simulink model "aerosonde_controlled"  (Simulink 7.7)
settings: Solver=ode3  StartTime=0.0  StopTime=200  FixedStep=20e-3  RelTol=1e-6
values from neighbouring files (symbols this model uses):
  aerosonde = aerosonde_data    [aerosonde_initialize.m]    (also in aerosonde_trimlin.m)
  chi_trim = 0    [aerosonde_initialize.m]
  eta_trim = -0.1    [aerosonde_initialize.m]
  euler_0 = [theta_trim; 0; 0]    [aerosonde_initialize.m]    (also in aerosonde_trimlin.m = xtrim(11:13))
  flap = 0    [aerosonde_initialize.m]
  fuel_0 = 2    [aerosonde_initialize.m]    (also in aerosonde_trimlin.m = xtrim(10))
  h_trim = 500    [aerosonde_initialize.m]
  ignition = 1    [aerosonde_initialize.m]
  Kari = 0.5    [aerosonde_initialize.m]
  Kd_Ye = 0.6    [aerosonde_initialize.m]
  Kd_Ze = -0.05    [aerosonde_initialize.m]
  Ki_phi = -0.1    [aerosonde_initialize.m]
  Ki_psi = 0.001    [aerosonde_initialize.m]
  Ki_theta = -0.8    [aerosonde_initialize.m]
  Ki_u = 0.15    [aerosonde_initialize.m]
  Ki_Ye = 0.0025    [aerosonde_initialize.m]
  Ki_Ze = -0.0001    [aerosonde_initialize.m]
  Kp_phi = -0.2    [aerosonde_initialize.m]
  Kp_psi = 0.7    [aerosonde_initialize.m]
  Kp_theta = -0.8    [aerosonde_initialize.m]
  Kp_u = 0.5    [aerosonde_initialize.m]
  Kp_Xe = 0.125    [aerosonde_initialize.m]
  Kp_Ye = 0.18    [aerosonde_initialize.m]
  Kp_Ze = -0.03    [aerosonde_initialize.m]
  Kphi_xi = -0.2    [aerosonde_initialize.m]
  Kq_eta = -0.28    [aerosonde_initialize.m]
  Kr_zeta = -0.25    [aerosonde_initialize.m]
  Ktheta_eta = -1    [aerosonde_initialize.m]
  latitude = 52.073105    [aerosonde_initialize.m]
  longitude = -000.616697    (= -0.616697)    [aerosonde_initialize.m]
  mixture = 13    [aerosonde_initialize.m]
  Omega_0 = 5000*pi/30    (= 523.598775598)    [aerosonde_initialize.m]    (also in aerosonde_trimlin.m = xtrim(14))
  position_0 = [0; 0; -h_trim]    [aerosonde_initialize.m]
  q_trim = 0    [aerosonde_initialize.m]
  rates_0 = [0; q_trim ; 0]    [aerosonde_initialize.m]    (also in aerosonde_trimlin.m = xtrim(7:9))
  tau_trim = 0.4    [aerosonde_initialize.m]
  theta_trim = 0    [aerosonde_initialize.m]
  Tr = 0.75    [aerosonde_initialize.m]
  Ue_VL = 25    [aerosonde_initialize.m]
  Ve_VL = 0    [aerosonde_initialize.m]
  velocity_0 = [23; 0; 0]    [aerosonde_initialize.m]    (also in aerosonde_trimlin.m = xtrim(1:3))
  We_VL = 0    [aerosonde_initialize.m]
  Xe0_VL = position_0(1)    [aerosonde_initialize.m]
  xi_trim = 0    [aerosonde_initialize.m]
  Ye0_VL = position_0(2)    [aerosonde_initialize.m]
  Ze0_VL = position_0(3)    [aerosonde_initialize.m]
  zeta_trim = 0    [aerosonde_initialize.m]
undefined symbols (not defined in the file or in its folder): Earth, F, m, MIL, rad, s, WGS84
libraries: aerolibasang x4, aerolibbdyn x3, aerolibfltsims x3, simulink_extras x3, aerolibwind2 x3, aerolibtransform2 x2, aerolibatmos2 x2, aerolibconvert2 x2, simulink x2, aerolibadyn x1, aerolib6dof2 x1, aerolibutil x1
(part 1 of 2)
settings Model: Creator=eh3081  LastModifiedBy=eh3081
settings DataIOCC: LimitDataPoints=off  SaveOutput=off  SignalLogging=off  SaveTime=off
settings OptimizationCC: InitFltsAndDblsToZero=on
settings DebuggingCC: SaveWithParameterizedLinksMsg=none  MultiTaskDSMMsg=warning  MultiTaskCondExecSysMsg=none  StrictBusMsg=Warning
settings RTWCC: IncludeERTFirstTime=on
settings GRTTargetCC: TargetFcnLib=ansi_tfl_tmw.mat

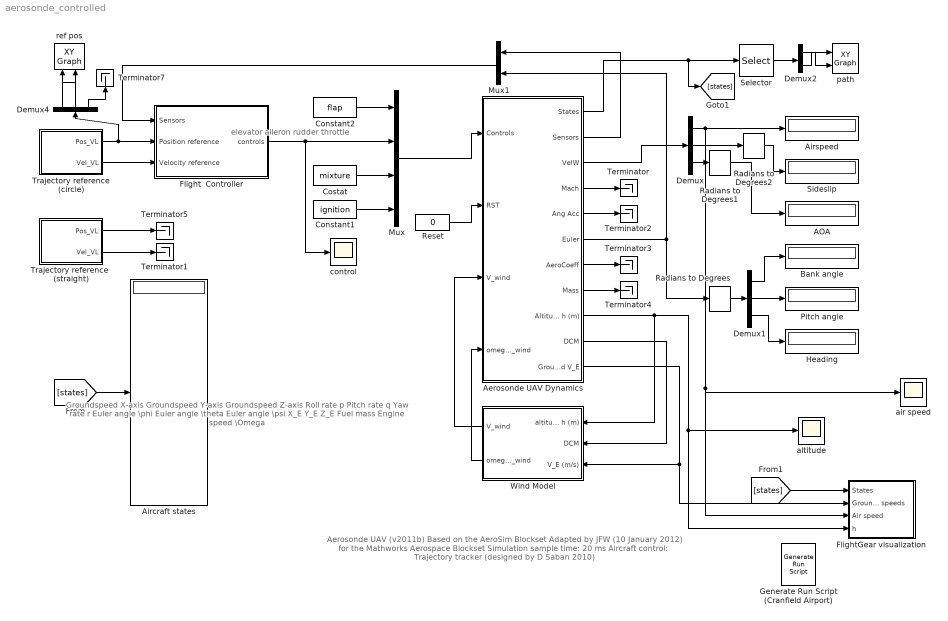
== system aerosonde_controlled ==
  note: Aerosonde UAV (v2011b)
      | Based on the AeroSim Blockset
      | Adapted by JFW (10 January 2012) for the Mathworks Aerospace Blockset
      | Simulation sample time: 20 ms
      | Aircraft control: Trajectory tracker (designed by D Saban 2010)
  note: Groundspeed X-axis
      | Groundspeed Y-axis
      | Groundspeed Z-axis
      | Roll rate p
      | Pitch rate q
      | Yaw rate r
      | Euler angle \phi
      | Euler angle \theta
      | Euler angle \psi
      | X_E
      | Y_E
      | Z_E
      | Fuel mass
      | Engine speed \Omega
  note: elevator
      | aileron
      | rudder
      | throttle
  AOA : Display
  Aerosonde UAV Dynamics : Subsystem  mask(6-DOF Aerosonde Model){as=aerosonde, Velocities0=velocity_0, Rates0=rates_0, Euler0=euler_0, Position0=position_0, Fuel0=fuel_0, Omega0=Omega_0, GndAlt=0}
      mask prompts: as "Aircraft configuration data:"; Velocities0 "Initial velocity in body axes [u,v,w]: (m/s)"; Rates0 "Initial body rotation rates [p,q,r]: (rad/s)"; Euler0 "Initial Euler orientation [roll, pitch, yaw]: (rad)"; Position0 "Initial position in inertial axes [Xe,Ye,Ze]: (m)"; Fuel0 "Initial fuel mass: (Kg)"; Omega0 "Initial engine speed: (rad/s)"; GndAlt "Ground altitude: (m)"
      mask help:
      | Nonlinear 6-DOF Aerosonde  model with equations of motion in
      | body frame.
      |
      | Version 2011a (18 February 2011)
      mask Help:
      | The block implements the 6-DOF nonlinear Aerosonde model. It is an adaptation of the model provided in the AeroSim blockset. Velocities are computed in body frame.
      | <P><B>Inputs:</B>
      | <LI>Controls = the 4x1 vector of aircraft controls [elevator aileron rudder throttle]. Aerodynamic controls are in radians, throttle is from 0 to 1.</LI>
      | <LI>RST = the integrator reset flag (0 or 1, all integrators on rising edge)
      | <LI>V_wind = the 3x1 vector of background wind speed components in navigation frame [North East Down]</LI>
      | <LI>omega_wind = the 3x1 vector of background wind angular rates in navigation frame [North East Down]</LI>
      | </P>
      | <P><B>Outputs:</B>
      | <LI>States = the 14x1 aircraft state vector [Velocities, Angular rates, Euler angles, Position, Fuel mass, Engine speed].</LI>
      | <LI>Sensors = the 15x1 vector of sensor outputs [GPS Position, GPS Groundspeed, Accelerometers, Gyros, Air data].</LI>
      | <LI>VelW = the 3x1 vector of aircraft velocity in wind axes [Airspeed, sideslip, angle of attack]</LI>
      | <LI>Mach = the Mach number</LI>
      | <LI>Ang Acc = the 3x1 vector of angular accelerations
      | <LI>Euler = the 3x1 vector of Euler angles (roll, pitch, yaw)</LI>
      | <LI>AeroCoeff = the 6x1 vector of aerodynamic coefficients [CD CY CL Cl Cm Cn]</LI>
      | <LI>Mass = the current aircraft mass</LI>
      | <LI>h = the aircraft altitude</LI>
      | </P>
      | <P><B>Parameters:</B>
      | <LI>Aircraft configuration data = structured varaible with aircraft data<BR>
      | obtain by  ``aerosonde=aerosonde_initialize'' for example</LI>
      | <LI>Initial velocities = the 3x1 vector of initial aircraft velocities in body axes [u v w]</LI>
      | <LI>Initial angular rates = the 3x1 vector of initial angular rates [p q r]</LI>
      | <LI>Initial attitude = the 3x1 vector of initial Euler angles [phi theta psi]</LI>
      | <LI>Initial position = the 3x1 vector of initial aircraft location [Lat Lon Alt]</LI>
      | <LI>Initial fuel mass = the initial quantity of fuel on-board the aircraft</LI>
      | <LI>Initial engine speed = the initial engine rotation speed</LI>
      | <LI>Ground altitude = the ground altitude at aircraft location</LI>
      | </P>
      | <P>
      | <I>Version 2010b (26 May 2010)</I>
      | </P>
  Aircraft states : Display
  Airspeed : Display
  Bank angle : Display
  Constant1 : Constant  Value=ignition
  Constant2 : Constant  Value=flap
  Costat : Constant  Value=mixture
  Demux : Demux  Outputs=3
  Demux1 : Demux  Outputs=3
  Demux2 : Demux  Outputs=2
  Demux4 : Demux  Outputs=3
  Flight  Controller : Subsystem
  FlightGear visualization : Subsystem  TreatAsAtomicUnit=on
  Generate Run Script (Cranfield Airport) : aerolibfltsims/Generate Run Script  SystemSampleTime=-1  OutputFileName=runfg.bat  FlightGearBaseDirectory=C:\Program Files\FlightGear 2.4.0  GeometryModelName=Aerosonde  DestinationPort=5502  AirportId=EGTC  RunwayId=3  InitialAltitude=h_trim*3.28083  InitialHeading=0  OffsetDistance=4.72  OffsetAzimuth=0  GenerateFile=off
  Heading : Display
  Mux : Mux  Inputs=[1 4 1 1]
  Mux1 : Mux  Inputs=[15 3]
  Pitch angle : Display
  Radians to Degrees : simulink_extras/Transformations/Radians to Degrees  SystemSampleTime=-1
  Radians to Degrees1 : simulink_extras/Transformations/Radians to Degrees  SystemSampleTime=-1
  Radians to Degrees2 : simulink_extras/Transformations/Radians to Degrees  SystemSampleTime=-1
  Reset : Constant  Value=0
  Selector : Selector  InputPortWidth=14  IndexOptions=Index vector (dialog)  Indices=[10 11]  OutputSizes=1
  Sideslip : Display
  Terminator{,1..5,7} (7 alike) : Terminator
  Trajectory reference (circle) : Subsystem
  Trajectory reference  (straight) : Subsystem
  Wind Model : Subsystem
  air speed : Scope
      settings: YMin=-2.5  YMax=25  SaveName=ScopeData2
  altitude : Scope
      settings: YMin=800  YMax=1025
  control : Scope
      settings: YMin=-0.1  YMax=1  SaveName=ScopeData5
  path : simulink/Sinks/XY Graph  SystemSampleTime=-1  xmin=-1000  xmax=1000  ymin=-1000  ymax=1000  st=-1
  ref pos : simulink/Sinks/XY Graph  SystemSampleTime=-1  xmin=-1000  xmax=1000  ymin=-1000  ymax=1000  st=-1
  wires:
  Reset/1 -> Aerosonde UAV Dynamics/2(RST)
  Aerosonde UAV Dynamics/1(States) -> Selector/1, [states]
  Aerosonde UAV Dynamics/6(Euler) -> Mux1/2, Radians to Degrees/1
  Demux/3 -> Radians to Degrees1/1
  Demux/2 -> Radians to Degrees2/1
  Demux/1 -> Airspeed/1, air speed/1, FlightGear visualization/3(Air speed)
  Radians to Degrees2/1 -> Sideslip/1
  Radians to Degrees1/1 -> AOA/1
  Radians to Degrees/1 -> Demux1/1
  Demux1/2 -> Pitch angle/1
  Demux1/3 -> Heading/1
  Demux1/1 -> Bank angle/1
  Aerosonde UAV Dynamics/3(VelW) -> Demux/1
  Wind Model/1(V_wind) -> Aerosonde UAV Dynamics/3(V_wind)
  Wind Model/2(omega_wind) -> Aerosonde UAV Dynamics/4(omega_wind)
  Aerosonde UAV Dynamics/9("Altitude h (m) ") -> Wind Model/1(altitude h (m)), altitude/1, FlightGear visualization/4(h)
  Aerosonde UAV Dynamics/10(DCM) -> Wind Model/2(DCM)
  Aerosonde UAV Dynamics/11(Groundspeed V_E) -> Wind Model/3(V_E (m/s)), FlightGear visualization/2(Ground speeds)
  Aerosonde UAV Dynamics/4(Mach) -> Terminator/1
  Aerosonde UAV Dynamics/5(Ang Acc) -> Terminator2/1
  Aerosonde UAV Dynamics/7(AeroCoeff) -> Terminator3/1
  Aerosonde UAV Dynamics/8(Mass) -> Terminator4/1
  Constant2/1 -> Mux/1
  Costat/1 -> Mux/3
  Constant1/1 -> Mux/4
  Mux/1 -> Aerosonde UAV Dynamics/1(Controls)
  Flight  Controller/1(controls) -> Mux/2, control/1
  Aerosonde UAV Dynamics/2(Sensors) -> Mux1/1
  Mux1/1 -> Flight  Controller/1(Sensors)
  Selector/1 -> Demux2/1
  [states] -> Aircraft states/1
  [states] -> FlightGear visualization/1(States)
  Trajectory reference  (straight)/2(Vel_VL) -> Terminator1/1
  Trajectory reference  (straight)/1(Pos_VL) -> Terminator5/1
  Trajectory reference (circle)/1(Pos_VL) -> Flight  Controller/2(Position reference), Demux4/1
  Trajectory reference (circle)/2(Vel_VL) -> Flight  Controller/3(Velocity reference)
  Demux2/2 -> path/1
  Demux2/1 -> path/2
  Demux4/2 -> ref pos/1
  Demux4/1 -> ref pos/2
  Demux4/3 -> Terminator7/1

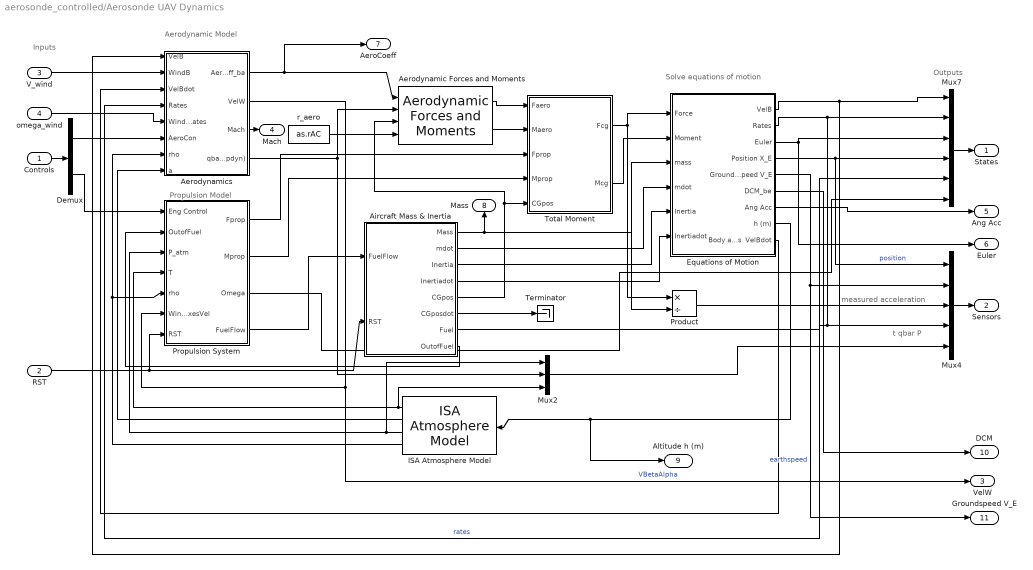
== system aerosonde_controlled/Aerosonde UAV Dynamics ==
  note: t qbar P
  note: measured acceleration
  note: Propulsion Model
  note: Aerodynamic Model
  note: Outputs
  note: Inputs
  note: Solve equations of motion
  Controls : Inport
  RST : Inport  Port=2
  V_wind : Inport  Port=3
  omega_wind : Inport  Port=4
  Aerodynamic Forces and Moments : aerolibadyn/Aerodynamic Forces and Moments   SystemSampleTime=-1  inputAxes=Body  outputForceAxes=Body  outputMomentAxes=Body  S=as.S  b=as.b  cbar=as.c
  Aerodynamics : Subsystem
  Aircraft Mass & Inertia : Subsystem
  Demux : Demux  Outputs=[4,3]
  Equations of Motion : Subsystem
  ISA Atmosphere Model : aerolibatmos2/ISA Atmosphere Model  SystemSampleTime=-1  custom=off  g=9.80665  gamma=1.4  R=287.0531  L=0.0065  h_trop=11000  h_strat=20000  rho0=1.225  P0=101325  T0=288.15
  Mux2 : Mux  Inputs=3
  Mux4 : Mux  Inputs=5
  Mux7 : Mux  Inputs=6
  Product : Product  Inputs=*/  RndMeth=Zero
  Propulsion System : Subsystem  mask(General-aviation propulsion system){OmegaIni=Omega0, RPM=as.RPM, MAP=as.MAP, FuelFlow=as.FuelFlow, Power=as.Power, Jeng=as.Jeng, J=as.J, CT=as.CT, CP=as.CP, Rprop=as.Rprop, Jprop=as.Jprop, TSL=as.TSL}
      mask prompts: OmegaIni "Initial engine speed:"; RPM "Engine RPM vector:"; MAP "Engine MAP vector:"; FuelFlow "Engine fuel flow look-up table:"; Power "Engine power look-up table:"; Jeng "Engine moment of inertia:"; J "Propeller advance ratio vector:"; CT "Propeller coefficient of thrust vector:"; CP "Propeller coefficient of power vector:"; Rprop "Propeller radius:"; Jprop "Propeller moment of inertia:"; TSL "Sea-level temperature:"
      mask help: The block models a general aviation propulsion system including a piston engine and a fixed-pitch propeller.
      mask Help:
      | The block provides a general aviation propulsion system using the AeroSim piston engine and fixed-pitch propeller models.
      | <P><B>Inputs:</B>
      | <LI>Control = the 3x1 engine control vector [Throttle Mixture Ignition]</LI>
      | <LI>OutofFuel = the out-of-fuel flag (0 or 1)</LI>
      | <LI>p = the static pressure at current altitude, in Pa</LI>
      | <LI>T = the air temperature at current altitude, in K</LI>
      | <LI>rho = the air density at current altitude, in kg/m^3</LI>
      | <LI>WindAxesVel = the 3x1 vector of body velocities in wind axes [Airspeed Sideslip Angle-of-attack] in [m/s rad rad]</LI>
      | <LI>RST = the integrator reset flag (rising edge)</LI>
      | </P>
      | <P><B>Output:</B>
      | <LI>Fprop = the 3x1 vector of propulsion system forces applied to the airframe, at the propeller hub location</LI>
      | <LI>Mprop = the 3x1 vector of propulsion system moments applied to the airframe</LI>
      | <LI>Omega = the engine shaft rotation speed, in rad/s</LI>
      | <LI>FuelFlow = the mass fuel flow, in kg/s</LI>
      | <LI>EngCoeff = the 5x1 engine coefficient vector [MAP Airflow Fuelflow BSFC Power] in [kPa kg/s kg/s g/(W*hr) W]</LI>
      | <LI>PropCoeff = the 3x1 propeller coefficient vector [J CT CP]</LI>
      | </P>
      | <P><B>Parameters:</B>
      | <LI>Initial engine speed = the initial value for the engine speed, in rad/s</LI>
      | <LI>RPM vector = the engine speed interpolation vector, in rpm</LI>
      | <LI>MAP vector = the manifold air pressure interpolation vector, in kPa</LI>
      | <LI>Fuel flow = the 2-D look-up table for fuel flow, as function of MAP and RPM, in g/hr</LI>
      | <LI>Power = the 2-D look-up table for power, as function of MAP and RPM, in W</LI>
      | <LI>Engine moment of inertia = the moment of inertia of the rotating engine parts (shaft)</LI>
      | <LI>Advance ratio = the advance ratio vector for interpolation</LI>
      | <LI>Coefficient of thrust = the coefficient of thrust vector for interpolation</LI>
      | <LI>Coefficient of power = the coefficient of power vector for interpolation</LI>
      | <LI>Radius = the propeller radius</LI>
      | <LI>Propeller moment of inertia = the moment of inertia of the propeller</LI>
      | <LI>Sea-level temperature = the ambient temperature for which the above engine look-up tables are given</LI>
      | </P>
  Terminator : Terminator
  Total Moment : Subsystem
  r_aero : Constant  Value=as.rAC
  States : Outport
  Sensors : Outport  Port=2
  VelW : Outport  Port=3
  Mach : Outport  Port=4
  Ang Acc : Outport  Port=5
  Euler : Outport  Port=6
  AeroCoeff : Outport  Port=7
  Mass : Outport  Port=8
  "Altitude h (m) " : Outport  Port=9
  DCM : Outport  Port=10
  Groundspeed V_E : Outport  Port=11
  wires:
  V_wind/1 -> Aerodynamics/2(WindB)
  omega_wind/1 -> Aerodynamics/5(WindRates)
  Equations of Motion/9(Body accns  VelBdot) -> Aerodynamics/3(VelBdot)
  Propulsion System/4(FuelFlow) -> Aircraft Mass & Inertia/1(FuelFlow)
  Product/1 -> Mux4/3
  Aircraft Mass & Inertia/6(CGposdot) -> Terminator/1
  Aircraft Mass & Inertia/4(Inertiadot) -> Equations of Motion/6(Inertiadot)
  Aircraft Mass & Inertia/3(Inertia) -> Equations of Motion/5(Inertia)
  Total Moment/1(Fcg) -> Product/1, Equations of Motion/1(Force)
  Aerodynamic Forces and Moments/2 -> Total Moment/2(Maero)
  Aerodynamic Forces and Moments/1 -> Total Moment/1(Faero)
  r_aero/1 -> Aerodynamic Forces and Moments/4
  Aircraft Mass & Inertia/2(mdot) -> Equations of Motion/4(mdot)
  Equations of Motion/8(h (m)) -> "Altitude h (m) "/1, ISA Atmosphere Model/1
  ISA Atmosphere Model/4 -> Propulsion System/5(rho), Aerodynamics/7(rho)
  ISA Atmosphere Model/3 -> Mux2/1, Propulsion System/3(P_atm)
  ISA Atmosphere Model/2 -> Aerodynamics/8("a ")
  ISA Atmosphere Model/1 -> Mux2/3, Propulsion System/4(T)
  Aerodynamics/1(AeroCoeff_ba) -> Aerodynamic Forces and Moments/1, AeroCoeff/1
  Aerodynamics/3(Mach) -> Mach/1
  Demux/1 -> Aerodynamics/6(AeroCon)
  Equations of Motion/4(Position X_E) -> Mux4/1, Mux7/4  "position"
  Equations of Motion/2(Rates) -> Mux7/2, Mux4/4, Aerodynamics/4(Rates)  "rates"
  Equations of Motion/1(VelB) -> Aerodynamics/1(VelB), Mux7/1
  Demux/2 -> Propulsion System/1(Eng Control)
  Mux7/1 -> States/1
  Mux4/1 -> Sensors/1
  Controls/1 -> Demux/1
  Equations of Motion/5(Groundspeed V_E) -> Groundspeed V_E/1, Mux4/2  "earthspeed"
  Aircraft Mass & Inertia/1(Mass) -> Product/2, Equations of Motion/3(mass), Mass/1
  Total Moment/2(Mcg) -> Equations of Motion/2(Moment)
  Aircraft Mass & Inertia/5(CGpos) -> Aerodynamic Forces and Moments/3, Total Moment/5(CGpos)
  Propulsion System/1(Fprop) -> Total Moment/3(Fprop)
  Propulsion System/2(Mprop) -> Total Moment/4(Mprop)
  Equations of Motion/6(DCM_be) -> DCM/1
  Aerodynamics/4(qbar (pdyn)) -> Aerodynamic Forces and Moments/2, Mux2/2
  Mux2/1 -> Mux4/5
  Aircraft Mass & Inertia/7(Fuel) -> Mux7/5
  Propulsion System/3(Omega) -> Mux7/6
  Aerodynamics/2(VelW) -> VelW/1, Propulsion System/6(WindAxesVel)  "VBetaAlpha"
  Aircraft Mass & Inertia/8(OutofFuel) -> Propulsion System/2(OutofFuel)
  RST/1 -> Aircraft Mass & Inertia/2(RST), Propulsion System/7(RST)
  Equations of Motion/7(Ang Acc) -> Ang Acc/1
  Equations of Motion/3(Euler) -> Mux7/3, Euler/1

== system aerosonde_controlled/Flight  Controller ==
  note: Flight Controller
      | for Aerosonde
      | (designed D Saban 2010)
  note: NOTE - this controller is trying to track
      | groundspeed which is difficult if wind
      | and turbulence are not light
      | NOTE that it is assumed that attitude is
      | measured and added to the sensor measurements
      | NOTE no sensor noise has been added
  note: complex
  Sensors : Inport
  Position reference : Inport  Port=2
  Velocity reference : Inport  Port=3
  Attitude controller : Subsystem
  Autopilot : Subsystem
  SAS : Subsystem
  Terminator : Terminator
  Trajectory tracker : Subsystem
  controls : Outport
  wires:
  Sensors/1 -> SAS/1(Sensors), Attitude controller/1(Sensors), Autopilot/1(Sensors), Trajectory tracker/1(Sensors)
  Attitude controller/1(demands) -> SAS/2(demands)  "eta_d xi_d tau_d"
  SAS/1(controls) -> controls/1  "elevator  aileron  rudder throttle"
  Autopilot/1(attitude_d) -> Attitude controller/2(attitude demands)  "theta_d phi_d tau_d"
  Trajectory tracker/2(psi_d (c)) -> Autopilot/3(psi_d(c))
  Position reference/1 -> Trajectory tracker/2(Pos_ref)
  Velocity reference/1 -> Trajectory tracker/3(Vel_ref)
  Trajectory tracker/4(errors) -> Terminator/1
  Trajectory tracker/1(h_d) -> Autopilot/2(h_d)
  Trajectory tracker/3(V_d) -> Autopilot/4(V_d)

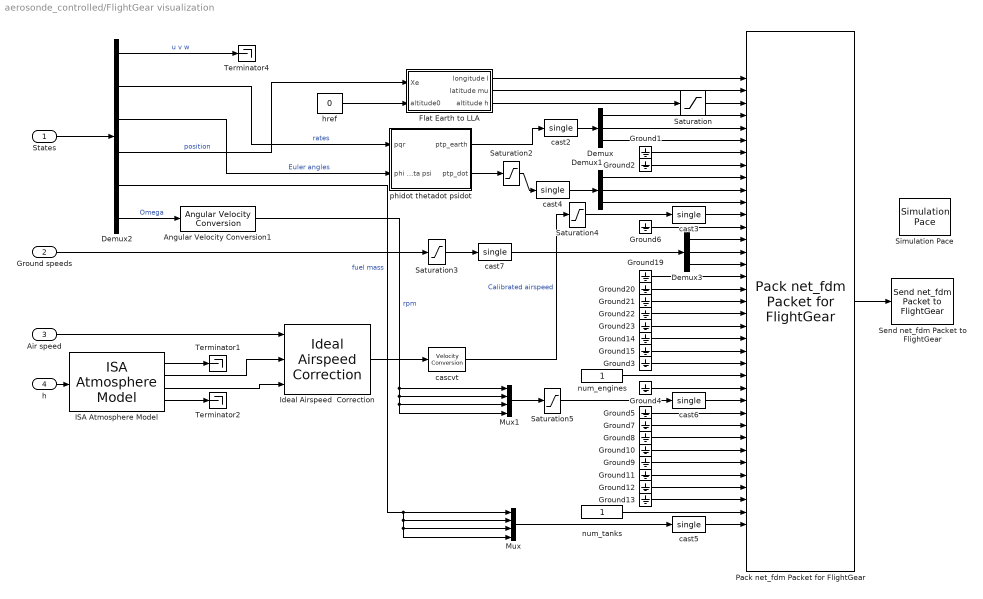
== system aerosonde_controlled/FlightGear visualization ==
  States : Inport
  Ground speeds : Inport  Port=2
  Air speed : Inport  Port=3
  h : Inport  Port=4
  Angular Velocity Conversion1 : aerolibconvert2/Angular Velocity Conversion  SystemSampleTime=-1  IU=rad/s  OU=rpm
  Demux : Demux  Outputs=3
  Demux1 : Demux  Outputs=3
  Demux2 : Demux  Outputs=[3 3 3 3 1 1]
  Demux3 : Demux  Outputs=3
  Flat Earth to LLA : Subsystem
  Ground{1..15,19..23} (20 alike) : Ground
  ISA Atmosphere Model : aerolibatmos2/ISA Atmosphere Model  SystemSampleTime=-1  custom=off  g=9.80665  gamma=1.4  R=287.0531  L=0.0065  h_trop=11000  h_strat=20000  rho0=1.225  P0=101325  T0=288.15
  Ideal Airspeed  Correction : aerolibasang/Ideal Airspeed Correction  SystemSampleTime=-1  units=Metric (MKS)  vel_in=TAS  vel_out_tas=CAS  vel_out_eas=CAS  vel_out_cas=TAS  action=Warning
  Mux : Mux
  Mux1 : Mux
  Pack net_fdm Packet for FlightGear : aerolibfltsims/Pack net_fdm Packet for FlightGear  FlightGearVersion=v2.0  ShowPositionAttitudeInputs=on  ShowVelocityAccelerationInputs=on  ShowControlSurfacePositionInputs=off  ShowEngineFuelInputs=on  ShowLandingGearInputs=off  ShowEnvironmentInputs=off  SampleTime=-1
      settings: AttributesFormatString=FG VERSION: %<FlightGearVersion>
  Saturation : Saturate  UpperLimit=1e8  LowerLimit=-1e5
  Saturation2 : Saturate  UpperLimit=1e3  LowerLimit=-1e3
  Saturation3 : Saturate  UpperLimit=1e4  LowerLimit=-1e4
  Saturation4 : Saturate  UpperLimit=1e4  LowerLimit=-1e4
  Saturation5 : Saturate  UpperLimit=1e6  LowerLimit=0
  Send net_fdm Packet to FlightGear : aerolibfltsims/Send net_fdm Packet to FlightGear  DestinationIpAddress=127.0.0.1  DestinationPort=5502  LocalIpPort=-1  varLen=off  SampleTime=-1
  Simulation Pace : aerolibanimutils/Simulation Pace  SimulationPace=1  SleepMode=MATLAB Thread  OutputPaceError=off  SampleTime=.2
      settings: AttributesFormatString=%<SimulationPace> sec/sec
  Terminator1 : Terminator
  Terminator2 : Terminator
  Terminator4 : Terminator
  cascvt : aerolibconvert/Velocity Conversion  SystemSampleTime=-1  IU=m/s  OU=kts
  cast{2..7} (6 alike) : DataTypeConversion  OutDataTypeStr=single  SaturateOnIntegerOverflow=on
  href : Constant  Value=0  VectorParams1D=off
  num_engines : Constant  OutDataTypeStr=uint32
  num_tanks : Constant  OutDataTypeStr=uint32
  phidot thetadot psidot : Subsystem
  wires:
  Pack net_fdm Packet for FlightGear/1 -> Send net_fdm Packet to FlightGear/1
  Ground4/1 -> Pack net_fdm Packet for FlightGear/26
  Ground3/1 -> Pack net_fdm Packet for FlightGear/24
  Demux1/3 -> Pack net_fdm Packet for FlightGear/11
  Demux1/2 -> Pack net_fdm Packet for FlightGear/10
  Demux1/1 -> Pack net_fdm Packet for FlightGear/9
  Ground2/1 -> Pack net_fdm Packet for FlightGear/8
  Ground1/1 -> Pack net_fdm Packet for FlightGear/7
  Demux/3 -> Pack net_fdm Packet for FlightGear/6
  Demux/2 -> Pack net_fdm Packet for FlightGear/5
  Demux/1 -> Pack net_fdm Packet for FlightGear/4
  Ground6/1 -> Pack net_fdm Packet for FlightGear/13
  ISA Atmosphere Model/2 -> Ideal Airspeed  Correction/2
  phidot thetadot psidot/2(ptp_dot) -> Saturation2/1
  phidot thetadot psidot/1(ptp_earth) -> cast2/1
  cast3/1 -> Pack net_fdm Packet for FlightGear/12
  Demux2/3 -> phidot thetadot psidot/2(phi theta psi)  "Euler angles"
  cascvt/1 -> Saturation4/1  "Calibrated airspeed"
  Ideal Airspeed  Correction/1 -> cascvt/1
  Ground15/1 -> Pack net_fdm Packet for FlightGear/23
  Ground14/1 -> Pack net_fdm Packet for FlightGear/22
  Ground23/1 -> Pack net_fdm Packet for FlightGear/21
  Ground22/1 -> Pack net_fdm Packet for FlightGear/20
  Ground21/1 -> Pack net_fdm Packet for FlightGear/19
  Ground20/1 -> Pack net_fdm Packet for FlightGear/18
  Ground19/1 -> Pack net_fdm Packet for FlightGear/17
  href/1 -> Flat Earth to LLA/2(altitude0)
  Flat Earth to LLA/3(altitude h) -> Saturation/1
  States/1 -> Demux2/1
  Demux2/2 -> phidot thetadot psidot/1(pqr)  "rates"
  Flat Earth to LLA/1(longitude l) -> Pack net_fdm Packet for FlightGear/1
  Flat Earth to LLA/2(latitude mu) -> Pack net_fdm Packet for FlightGear/2
  Demux2/4 -> Flat Earth to LLA/1(Xe)  "position"
  Demux3/1 -> Pack net_fdm Packet for FlightGear/14
  Demux3/2 -> Pack net_fdm Packet for FlightGear/15
  Demux3/3 -> Pack net_fdm Packet for FlightGear/16
  Ground speeds/1 -> Saturation3/1
  num_engines/1 -> Pack net_fdm Packet for FlightGear/25
  cast2/1 -> Demux/1
  cast4/1 -> Demux1/1
  Demux2/1 -> Terminator4/1  "u v w"
  cast5/1 -> Pack net_fdm Packet for FlightGear/37
  cast6/1 -> Pack net_fdm Packet for FlightGear/27
  Ground5/1 -> Pack net_fdm Packet for FlightGear/28
  Ground7/1 -> Pack net_fdm Packet for FlightGear/29
  Ground8/1 -> Pack net_fdm Packet for FlightGear/30
  Ground10/1 -> Pack net_fdm Packet for FlightGear/31
  Ground9/1 -> Pack net_fdm Packet for FlightGear/32
  Ground11/1 -> Pack net_fdm Packet for FlightGear/33
  Ground12/1 -> Pack net_fdm Packet for FlightGear/34
  Ground13/1 -> Pack net_fdm Packet for FlightGear/35
  num_tanks/1 -> Pack net_fdm Packet for FlightGear/36
  Air speed/1 -> Ideal Airspeed  Correction/1
  ISA Atmosphere Model/1 -> Terminator1/1
  ISA Atmosphere Model/4 -> Terminator2/1
  ISA Atmosphere Model/3 -> Ideal Airspeed  Correction/3
  h/1 -> ISA Atmosphere Model/1
  Demux2/5 -> Mux/1, Mux/2, Mux/3, Mux/4  "fuel mass"
  Mux/1 -> cast5/1
  Demux2/6 -> Angular Velocity Conversion1/1  "Omega"
  Mux1/1 -> Saturation5/1
  cast7/1 -> Demux3/1
  Angular Velocity Conversion1/1 -> Mux1/1, Mux1/2, Mux1/3, Mux1/4  "rpm"
  Saturation/1 -> Pack net_fdm Packet for FlightGear/3
  Saturation2/1 -> cast4/1
  Saturation3/1 -> cast7/1
  Saturation4/1 -> cast3/1
  Saturation5/1 -> cast6/1

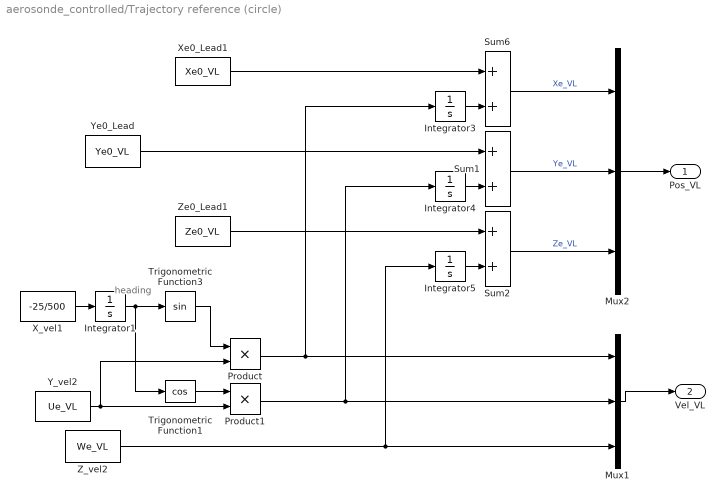
== system aerosonde_controlled/Trajectory reference (circle) ==
  note: heading
  Integrator{1,3..5} (4 alike) : Integrator
  Mux1 : Mux  Inputs=3
  Mux2 : Mux  Inputs=3
  Product : Product  RndMeth=Zero
  Product1 : Product  RndMeth=Zero
  Sum1 : Sum
  Sum2 : Sum
  Sum6 : Sum
  Trigonometric Function1 : Trigonometry  Operator=cos
  Trigonometric Function3 : Trigonometry
  X_vel1 : Constant  Value=-25/500
  Xe0_Lead1 : Constant  Value=Xe0_VL
  Y_vel2 : Constant  Value=Ue_VL
  Ye0_Lead : Constant  Value=Ye0_VL
  Z_vel2 : Constant  Value=We_VL
  Ze0_Lead1 : Constant  Value=Ze0_VL
  Pos_VL : Outport
  Vel_VL : Outport  Port=2
  wires:
  Trigonometric Function1/1 -> Product1/1
  Integrator1/1 -> Trigonometric Function3/1, Trigonometric Function1/1
  X_vel1/1 -> Integrator1/1
  Trigonometric Function3/1 -> Product/1
  Product1/1 -> Integrator4/1, Mux1/2
  Product/1 -> Integrator3/1, Mux1/1
  Z_vel2/1 -> Integrator5/1, Mux1/3
  Mux1/1 -> Vel_VL/1
  Y_vel2/1 -> Product1/2, Product/2
  Ye0_Lead/1 -> Sum1/1
  Xe0_Lead1/1 -> Sum6/1
  Ze0_Lead1/1 -> Sum2/1
  Integrator3/1 -> Sum6/2
  Integrator4/1 -> Sum1/2
  Integrator5/1 -> Sum2/2
  Mux2/1 -> Pos_VL/1
  Sum2/1 -> Mux2/3  "Ze_VL"
  Sum1/1 -> Mux2/2  "Ye_VL"
  Sum6/1 -> Mux2/1  "Xe_VL"

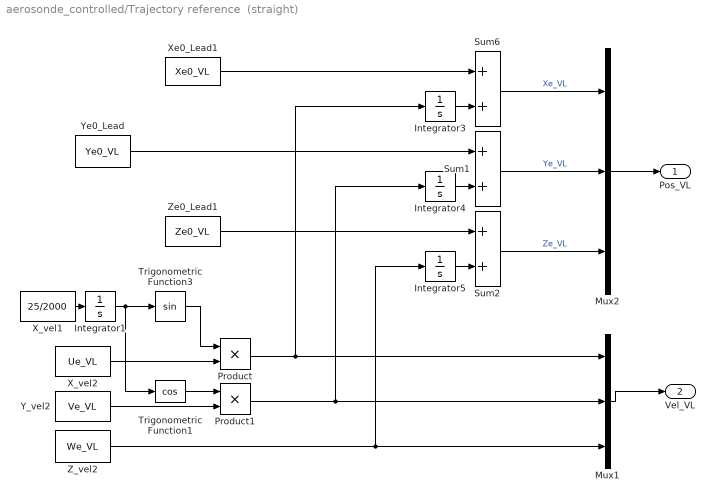
== system aerosonde_controlled/Trajectory reference  (straight) ==
  Integrator{1,3..5} (4 alike) : Integrator
  Mux1 : Mux  Inputs=3
  Mux2 : Mux  Inputs=3
  Product : Product  RndMeth=Zero
  Product1 : Product  RndMeth=Zero
  Sum1 : Sum
  Sum2 : Sum
  Sum6 : Sum
  Trigonometric Function1 : Trigonometry  Operator=cos
  Trigonometric Function3 : Trigonometry
  X_vel1 : Constant  Value=25/2000
  X_vel2 : Constant  Value=Ue_VL
  Xe0_Lead1 : Constant  Value=Xe0_VL
  Y_vel2 : Constant  Value=Ve_VL
  Ye0_Lead : Constant  Value=Ye0_VL
  Z_vel2 : Constant  Value=We_VL
  Ze0_Lead1 : Constant  Value=Ze0_VL
  Pos_VL : Outport
  Vel_VL : Outport  Port=2
  wires:
  Sum6/1 -> Mux2/1  "Xe_VL"
  Sum1/1 -> Mux2/2  "Ye_VL"
  Sum2/1 -> Mux2/3  "Ze_VL"
  Mux2/1 -> Pos_VL/1
  Integrator5/1 -> Sum2/2
  Integrator4/1 -> Sum1/2
  Integrator3/1 -> Sum6/2
  Ze0_Lead1/1 -> Sum2/1
  Xe0_Lead1/1 -> Sum6/1
  Ye0_Lead/1 -> Sum1/1
  X_vel2/1 -> Product/2
  Y_vel2/1 -> Product1/2
  Mux1/1 -> Vel_VL/1
  Z_vel2/1 -> Mux1/3, Integrator5/1
  Product/1 -> Mux1/1, Integrator3/1
  Product1/1 -> Mux1/2, Integrator4/1
  Trigonometric Function3/1 -> Product/1
  X_vel1/1 -> Integrator1/1
  Integrator1/1 -> Trigonometric Function3/1, Trigonometric Function1/1
  Trigonometric Function1/1 -> Product1/1

== system aerosonde_controlled/Wind Model ==
  note: Wind Models
  altitude h (m) : Inport
  DCM : Inport  Port=2
  V_E (m/s) : Inport  Port=3
  Dot Product : DotProduct  SaturateOnIntegerOverflow=on  OutDataTypeStr=Inherit: Inherit via internal rule
  Dryden Wind Turbulence Model  (Continuous (+q +r)) : aerolibwind2/Dryden Wind Turbulence Model  (Continuous (+q -r))  SystemSampleTime=-1  units=Metric (MKS)  spec=MIL-F-8785C  model=Continuous Von Karman (+q -r)  W20=0  Wdeg=90  TurbProb=2x10^-1  L_high=533.4  Wingspan=aerosonde.b  ts=0.02  Seed=[23341 23342 23343 23344]  T_on=on
  Horizontal Wind Model : aerolibwind2/Horizontal Wind Model  SystemSampleTime=-1  units=Metric (MKS)  Vw_source=Internal  Vwind=0  W_source=Internal  Wdeg=-60
  Sum : Sum  Inputs=+++  SaturateOnIntegerOverflow=on  InputSameDT=on  OutDataTypeStr=Inherit: Same as first input
  V : Math  Operator=sqrt  SaturateOnIntegerOverflow=on
  Wind Shear Model : aerolibwind2/Wind Shear Model  SystemSampleTime=-1  units=Metric (MKS)  phase=Category C - Terminal Flight Phase  W_20=0  Wdeg=0
  ground speed1 : Scope
      settings: YMin=20.75  YMax=26.25  SaveName=ScopeData4
  V_wind : Outport
  omega_wind : Outport  Port=2
  wires:
  Wind Shear Model/1 -> Sum/1
  Horizontal Wind Model/1 -> Sum/2
  altitude h (m)/1 -> Wind Shear Model/1, Dryden Wind Turbulence Model  (Continuous (+q +r))/1
  DCM/1 -> Horizontal Wind Model/1, Wind Shear Model/2, Dryden Wind Turbulence Model  (Continuous (+q +r))/3
  Sum/1 -> V_wind/1
  Dryden Wind Turbulence Model  (Continuous (+q +r))/2 -> omega_wind/1
  Dot Product/1 -> V/1
  V_E (m/s)/1 -> Dot Product/1, Dot Product/2
  Dryden Wind Turbulence Model  (Continuous (+q +r))/1 -> Sum/3
  V/1 -> Dryden Wind Turbulence Model  (Continuous (+q +r))/2, ground speed1/1

== system aerosonde_controlled/Aerosonde UAV Dynamics/Aerodynamics ==
  note: Aerodynamic Model
  note: Aerodynamic Coefficients
  note: Aerodynamic Parameters
  note: Outputs
  note: Inputs
  VelB : Inport  PortDimensions=[3 1]
  WindB : Inport  Port=2  PortDimensions=[3 1]
  VelBdot : Inport  Port=3
  Rates : Inport  Port=4  PortDimensions=[3 1]
  WindRates : Inport  Port=5  PortDimensions=[3 1]
  AeroCon : Inport  Port=6  PortDimensions=[4 1]
  rho : Inport  Port=7  PortDimensions=1
  "a " : Inport  Port=8  PortDimensions=1
  Force Coefficients : Subsystem
  Moment Coefficients : Subsystem
  Mux : Mux  Inputs=2
  Sum : Sum  Inputs=|+-  SaturateOnIntegerOverflow=on  InputSameDT=on  OutDataTypeStr=Inherit: Same as first input
  Wind-axes Velocities : Subsystem
  AeroCoeff_ba : Outport
  VelW : Outport  Port=2
  Mach : Outport  Port=3
  qbar (pdyn) : Outport  Port=4
  wires:
  VelBdot/1 -> Wind-axes Velocities/5(VelBdot)
  Wind-axes Velocities/4(alphadot) -> Force Coefficients/3(AlphaDot), Moment Coefficients/3(AlphaDot)
  WindB/1 -> Wind-axes Velocities/2(WindB)
  Mux/1 -> AeroCoeff_ba/1
  Moment Coefficients/1("[-Cl, Cm, -Cn]") -> Mux/2
  Force Coefficients/1("[-CD, CY, -CL]") -> Mux/1
  rho/1 -> Wind-axes Velocities/4(rho)
  VelB/1 -> Wind-axes Velocities/1(VelB)
  "a "/1 -> Wind-axes Velocities/3(a)  "speed of sound"
  Wind-axes Velocities/1(VBetaAlpha) -> Moment Coefficients/1(VBetaAlpha), VelW/1, Force Coefficients/1(VBetaAlpha)
  AeroCon/1 -> Moment Coefficients/2(Control), Force Coefficients/2(Control)
  Wind-axes Velocities/2(Mach) -> Moment Coefficients/5(Mach), Force Coefficients/5(Mach), Mach/1
  Wind-axes Velocities/3(qbar (pdyn)) -> qbar (pdyn)/1
  Rates/1 -> Sum/1
  WindRates/1 -> Sum/2
  Sum/1 -> Moment Coefficients/4(AngularRates), Force Coefficients/4(AngularRates)  "pqr"

== system aerosonde_controlled/Aerosonde UAV Dynamics/Aircraft Mass & Inertia ==
  note: Compute current aircraft mass
  FuelFlow : Inport  PortDimensions=1
  RST : Inport  Port=2  PortDimensions=1
  ChSign : Gain  Gain=-1  SaturateOnIntegerOverflow=on  OutDataTypeStr=Inherit: Same as input  ParamDataTypeStr=Inherit: Same as input
  Estimate Center of Gravity : aerolibbdyn/Estimate Center of Gravity  SystemSampleTime=-1  fmass=as.mgross  emass=as.mempty  fcg=as.CGgross  ecg=as.CGempty
  Estimate Inertia Tensor : aerolibbdyn/Estimate Inertia Tensor  SystemSampleTime=-1  fmass=as.mgross  emass=as.mempty  fI=as.J_gross  eI=as.J_empty
  Fuel Integrator : Integrator  ExternalReset=rising  InitialCondition=Fuel0  LimitOutput=on  UpperSaturationLimit=as.mgross-as.mempty  LowerSaturationLimit=0
  Mass empty : Constant  Value=as.mempty
  Relational Operator : RelationalOperator  Operator===  InputSameDT=on
  Sum : Sum  Inputs=|++  SaturateOnIntegerOverflow=on  InputSameDT=on  OutDataTypeStr=Inherit: Same as first input
  Mass : Outport
  mdot : Outport  Port=2
  Inertia : Outport  Port=3
  Inertiadot : Outport  Port=4
  CGpos : Outport  Port=5
  CGposdot : Outport  Port=6
  Fuel : Outport  Port=7
  OutofFuel : Outport  Port=8
  wires:
  Estimate Center of Gravity/2 -> CGposdot/1
  Estimate Center of Gravity/1 -> CGpos/1
  Estimate Inertia Tensor/2 -> Inertiadot/1
  Estimate Inertia Tensor/1 -> Inertia/1
  Sum/1 -> Relational Operator/1, Estimate Center of Gravity/1, Estimate Inertia Tensor/1, Mass/1
  Mass empty/1 -> Sum/2, Relational Operator/2
  Fuel Integrator/1 -> Sum/1, Fuel/1
  RST/1 -> Fuel Integrator/2
  ChSign/1 -> Estimate Center of Gravity/2, Estimate Inertia Tensor/2, mdot/1, Fuel Integrator/1
  FuelFlow/1 -> ChSign/1
  Relational Operator/1 -> OutofFuel/1

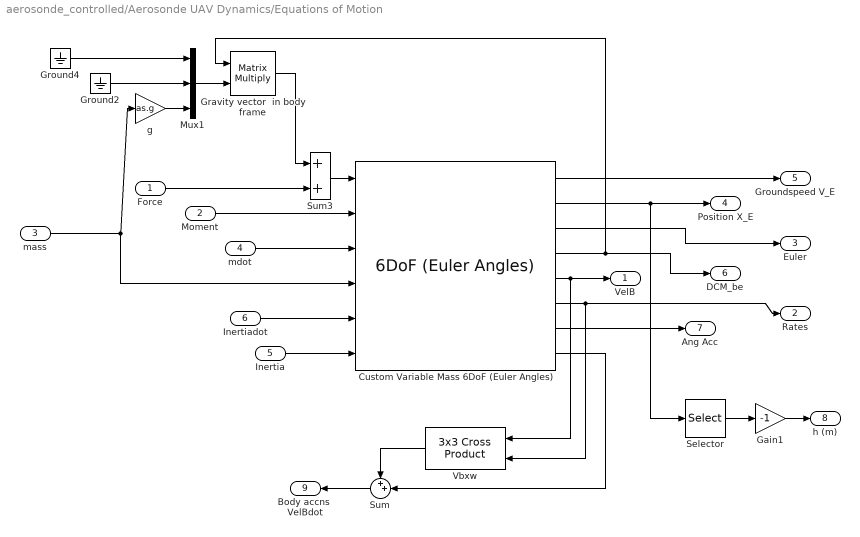
== system aerosonde_controlled/Aerosonde UAV Dynamics/Equations of Motion ==
  Force : Inport  PortDimensions=3
  Moment : Inport  Port=2  PortDimensions=3
  mass : Inport  Port=3  PortDimensions=1
  mdot : Inport  Port=4  PortDimensions=1
  Inertia : Inport  Port=5  PortDimensions=[3,3]
  Inertiadot : Inport  Port=6  PortDimensions=[3,3]
  Custom Variable Mass 6DoF (Euler Angles) : aerolib6dof2/6DoF (Euler Angles)  SystemSampleTime=-1  units=Metric (MKS)  mtype=Custom Variable  rep=Euler Angles  xme_0=Position0  Vm_0=Velocities0  eul_0=Euler0  pm_0=Rates0  mass_0=1.0  mass_e=0  mass_f=0  inertia=eye(3)  inertia_e=eye(3)  inertia_f=eye(3)  k_quat=1.0
  Gain1 : Gain  Gain=-1
  "Gravity vector  in body frame " : Product  Multiplication=Matrix(*)  SaturateOnIntegerOverflow=on  InputSameDT=on  OutDataTypeStr=Inherit: Same as first input
  Ground2 : Ground
  Ground4 : Ground
  Mux1 : Mux  Inputs=3
  Selector : Selector  InputPortWidth=3  IndexOptions=Index vector (dialog)  Indices=3  OutputSizes=1
  Sum : Sum  Inputs=++|  SaturateOnIntegerOverflow=on
  Sum3 : Sum  SaturateOnIntegerOverflow=on  InputSameDT=on  OutDataTypeStr=Inherit: Same as first input
  Vbxw : aerolibutil/3x3 Cross Product  SystemSampleTime=-1
  g : Gain  Gain=as.g
  VelB : Outport
  Rates : Outport  Port=2
  Euler : Outport  Port=3
  Position X_E : Outport  Port=4
  Groundspeed V_E : Outport  Port=5
  DCM_be : Outport  Port=6
  Ang Acc : Outport  Port=7
  h (m) : Outport  Port=8
  Body accns  VelBdot : Outport  Port=9
  wires:
  Vbxw/1 -> Sum/1
  Sum/1 -> Body accns  VelBdot/1
  Custom Variable Mass 6DoF (Euler Angles)/8 -> Sum/2
  Custom Variable Mass 6DoF (Euler Angles)/7 -> Ang Acc/1
  Custom Variable Mass 6DoF (Euler Angles)/6 -> Vbxw/2, Rates/1
  Inertia/1 -> Custom Variable Mass 6DoF (Euler Angles)/6
  mdot/1 -> Custom Variable Mass 6DoF (Euler Angles)/3
  Inertiadot/1 -> Custom Variable Mass 6DoF (Euler Angles)/5
  Gain1/1 -> h (m)/1
  Selector/1 -> Gain1/1
  Sum3/1 -> Custom Variable Mass 6DoF (Euler Angles)/1
  g/1 -> Mux1/3
  "Gravity vector  in body frame "/1 -> Sum3/1
  Custom Variable Mass 6DoF (Euler Angles)/3 -> Euler/1
  Custom Variable Mass 6DoF (Euler Angles)/2 -> Selector/1, Position X_E/1
  Custom Variable Mass 6DoF (Euler Angles)/1 -> Groundspeed V_E/1
  Custom Variable Mass 6DoF (Euler Angles)/5 -> Vbxw/1, VelB/1
  Ground4/1 -> Mux1/1
  Ground2/1 -> Mux1/2
  mass/1 -> Custom Variable Mass 6DoF (Euler Angles)/4, g/1
  Custom Variable Mass 6DoF (Euler Angles)/4 -> DCM_be/1, "Gravity vector  in body frame "/1
  Mux1/1 -> "Gravity vector  in body frame "/2
  Force/1 -> Sum3/2
  Moment/1 -> Custom Variable Mass 6DoF (Euler Angles)/2

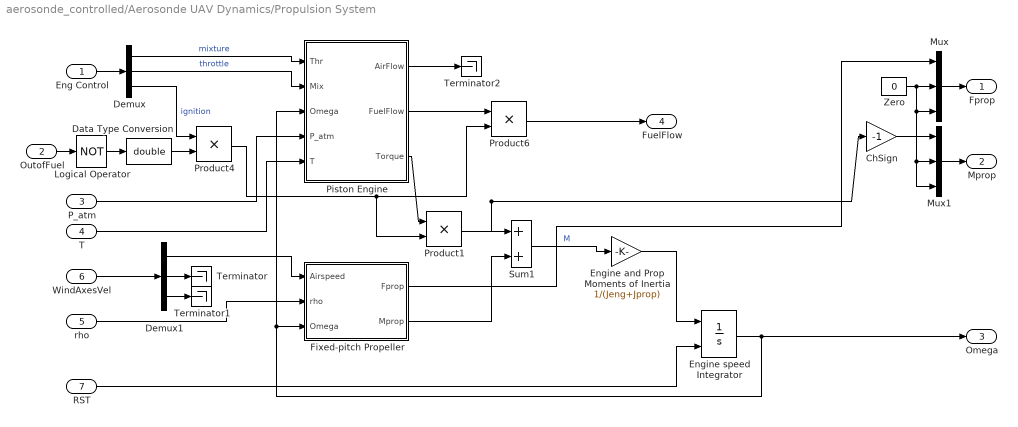
== system aerosonde_controlled/Aerosonde UAV Dynamics/Propulsion System ==
  Eng Control : Inport  PortDimensions=[3 1]
  OutofFuel : Inport  Port=2  PortDimensions=1
  P_atm : Inport  Port=3  OutDataTypeStr=double  PortDimensions=1
  T : Inport  Port=4  OutDataTypeStr=double  PortDimensions=1
  rho : Inport  Port=5  OutDataTypeStr=double  PortDimensions=1
  WindAxesVel : Inport  Port=6  PortDimensions=[3 1]
  RST : Inport  Port=7  OutDataTypeStr=double  PortDimensions=1
  ChSign : Gain  Gain=-1  SaturateOnIntegerOverflow=on  OutDataTypeStr=Inherit: Same as input  ParamDataTypeStr=Inherit: Same as input
  Data Type Conversion : DataTypeConversion  OutDataTypeStr=double  SaturateOnIntegerOverflow=on  RndMeth=Zero
  Demux : Demux  Outputs=3
  Demux1 : Demux  Outputs=3
  Engine and Prop Moments of Inertia : Gain  Gain=1/(Jeng+Jprop)  SaturateOnIntegerOverflow=on  OutDataTypeStr=Inherit: Same as input  ParamDataTypeStr=Inherit: Same as input
  Engine speed Integrator : Integrator  ExternalReset=rising  InitialCondition=OmegaIni  LimitOutput=on  LowerSaturationLimit=0
  Fixed-pitch Propeller : Subsystem
  Logical Operator : Logic  Operator=NOT
  Mux : Mux  Inputs=3
  Mux1 : Mux  Inputs=3
  Piston Engine : Subsystem  mask(Piston Engine){RPM=RPM, MAP=MAP, fflow=FuelFlow, Power=Power, TSL=TSL}
      mask prompts: RPM "RPM vector:"; MAP "MAP vector:"; fflow "Fuel flow 2-D look-up table:"; Power "Power 2-D look-up table:"; TSL "Sea-level temperature:"
      mask help: The piston engine model computes the engine parameters at current throttle setting, engine rpm, and altitude.
      mask Help:
      | The block provides a piston engine model based on look-up tables for manifold pressure, engine speed (rpm), fuel flow and power.
      | <P><B>Inputs:</B>
      | <LI>Thr = the throttle command (as a fraction of atmospheric pressure)</LI>
      | <LI>Mix = the air to fuel mixture ratio</LI>
      | <LI>Omega = the engine shaft rotation speed</LI>
      | <LI>p = the atmospheric pressure, in Pa</LI>
      | <LI>T = the atmospheric temperature, in K</LI>
      | </P>
      | <P><B>Output:</B>
      | <LI>MAP = the manifold air pressure, in kPa</LI>
      | <LI>AirFlow = the mass air flow, in kg/s</LI>
      | <LI>FuelFlow = the mass fuel flow, in kg/s</LI>
      | <LI>BSFC = the brake-specific fuel consumption, in g/(W*hr)</LI>
      | <LI>Power = the engine power, in W</LI>
      | <LI>Torque = the engine shaft torque, in N*m</LI>
      | </P>
      | <P><B>Parameters:</B>
      | <LI>RPM vector = the engine speed interpolation vector, in rpm</LI>
      | <LI>MAP vector = the manifold air pressure interpolation vector, in kPa</LI>
      | <LI>Fuel flow = the 2-D look-up table for fuel flow, as function of MAP and RPM, in g/hr</LI>
      | <LI>Power = the 2-D look-up table for power, as function of MAP and RPM, in W</LI>
      | <LI>Sea-level temperature = the ambient temperature for which the above engine look-up tables are given</LI>
      | </P>
  Product1 : Product  SaturateOnIntegerOverflow=on  InputSameDT=on  OutDataTypeStr=Inherit: Same as first input
  Product4 : Product  SaturateOnIntegerOverflow=on  InputSameDT=on  OutDataTypeStr=Inherit: Same as first input
  Product6 : Product  SaturateOnIntegerOverflow=on  InputSameDT=on  OutDataTypeStr=Inherit: Same as first input
  Sum1 : Sum  SaturateOnIntegerOverflow=on  InputSameDT=on  OutDataTypeStr=Inherit: Same as first input
  Terminator : Terminator
  Terminator1 : Terminator
  Terminator2 : Terminator
  Zero : Constant  Value=0
  Fprop : Outport
  Mprop : Outport  Port=2
  Omega : Outport  Port=3
  FuelFlow : Outport  Port=4
  wires:
  Piston Engine/1(AirFlow) -> Terminator2/1
  Product6/1 -> FuelFlow/1
  Piston Engine/2(FuelFlow) -> Product6/1
  Engine and Prop Moments of Inertia/1 -> Engine speed Integrator/1
  T/1 -> Piston Engine/5(T)
  P_atm/1 -> Piston Engine/4(P_atm)
  Demux/2 -> Piston Engine/2(Mix)  "throttle"
  Demux/1 -> Piston Engine/1(Thr)  "mixture"
  Demux/3 -> Product4/1  "ignition"
  Logical Operator/1 -> Data Type Conversion/1
  Mux1/1 -> Mprop/1
  Mux/1 -> Fprop/1
  ChSign/1 -> Mux1/1
  Fixed-pitch Propeller/1(Fprop) -> Mux/1
  Zero/1 -> Mux1/2, Mux1/3, Mux/3, Mux/2
  Piston Engine/3(Torque) -> Product1/1
  Engine speed Integrator/1 -> Omega/1, Piston Engine/3(Omega), Fixed-pitch Propeller/3(Omega)
  RST/1 -> Engine speed Integrator/2
  Sum1/1 -> Engine and Prop Moments of Inertia/1  "M"
  Fixed-pitch Propeller/2(Mprop) -> Sum1/2
  Product1/1 -> ChSign/1, Sum1/1
  Product4/1 -> Product1/2, Product6/2
  OutofFuel/1 -> Logical Operator/1
  rho/1 -> Fixed-pitch Propeller/2(rho)
  Demux1/1 -> Fixed-pitch Propeller/1(Airspeed)
  Demux1/3 -> Terminator1/1
  Demux1/2 -> Terminator/1
  WindAxesVel/1 -> Demux1/1
  Eng Control/1 -> Demux/1
  Data Type Conversion/1 -> Product4/2

== system aerosonde_controlled/Aerosonde UAV Dynamics/Total Moment ==
  note: Sum forces and moments
  note: Total moments at CG location
  Faero : Inport  PortDimensions=3
  Maero : Inport  Port=2  PortDimensions=3
  Fprop : Inport  Port=3  PortDimensions=3
  Mprop : Inport  Port=4  PortDimensions=3
  CGpos : Inport  Port=5  PortDimensions=3
  Moments about CG  due to Propulsion   Forces : aerolibbdyn/Moments about CG  due to Forces  SystemSampleTime=-1
  Sum1 : Sum  Inputs=+++  SaturateOnIntegerOverflow=on  InputSameDT=on  OutDataTypeStr=Inherit: Same as first input
  Total forces  (excluding g) : Sum  SaturateOnIntegerOverflow=on  InputSameDT=on  OutDataTypeStr=Inherit: Same as first input
  r_prop : Constant  Value=as.rHub  OutDataTypeStr=double
  Fcg : Outport
  Mcg : Outport  Port=2
  wires:
  Maero/1 -> Sum1/2
  Moments about CG  due to Propulsion   Forces/1 -> Sum1/1
  Total forces  (excluding g)/1 -> Fcg/1
  Faero/1 -> Total forces  (excluding g)/1
  Fprop/1 -> Total forces  (excluding g)/2, Moments about CG  due to Propulsion   Forces/1
  Mprop/1 -> Sum1/3
  Sum1/1 -> Mcg/1
  r_prop/1 -> Moments about CG  due to Propulsion   Forces/3
  CGpos/1 -> Moments about CG  due to Propulsion   Forces/2

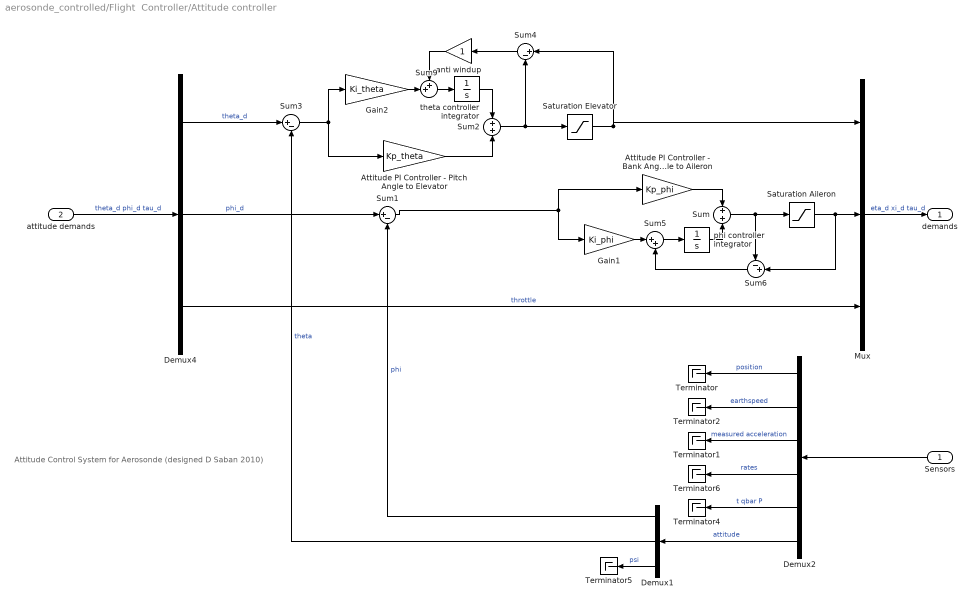
== system aerosonde_controlled/Flight  Controller/Attitude controller ==
  note: Attitude Control System
      | for Aerosonde
      | (designed D Saban 2010)
  Sensors : Inport
  attitude demands : Inport  Port=2
  Attitude PI Controller - Bank Angle to Aileron : Gain  Gain=Kp_phi
  Attitude PI Controller - Pitch Angle to Elevator : Gain  Gain=Kp_theta
  Demux1 : Demux  Outputs=3
  Demux2 : Demux  Outputs=[3 3 3 3 3 3]
  Demux4 : Demux  Outputs=3
  Gain1 : Gain  Gain=Ki_phi
  Gain2 : Gain  Gain=Ki_theta
  Mux : Mux  Inputs=3
  Saturation Aileron : Saturate  UpperLimit=20*pi/180  LowerLimit=-20*pi/180  ZeroCross=off
  Saturation Elevator : Saturate  UpperLimit=20*pi/180  LowerLimit=-20*pi/180  ZeroCross=off
  Sum : Sum  Inputs=+|+
  Sum1 : Sum  Inputs=|+-
  Sum2 : Sum  Inputs=+|+
  Sum3 : Sum  Inputs=|+-
  Sum4 : Sum  Inputs=|+-
  Sum5 : Sum  Inputs=|++
  Sum6 : Sum  Inputs=-+|
  Sum9 : Sum  Inputs=++|
  Terminator{,1..2,4..6} (6 alike) : Terminator
  anti windup : Gain
  phi controller integrator : Integrator  InitialCondition=xi_trim
  theta controller integrator : Integrator  InitialCondition=eta_trim + Ktheta_eta*theta_trim + Kq_eta*q_trim
  demands : Outport
  wires:
  Sum1/1 -> Attitude PI Controller - Bank Angle to Aileron/1, Gain1/1
  Demux4/2 -> Sum1/1  "phi_d"
  Sum3/1 -> Gain2/1, Attitude PI Controller - Pitch Angle to Elevator/1
  theta controller integrator/1 -> Sum2/1
  Attitude PI Controller - Pitch Angle to Elevator/1 -> Sum2/2
  Gain2/1 -> Sum9/2
  Sum9/1 -> theta controller integrator/1
  Sum2/1 -> Saturation Elevator/1, Sum4/2
  Saturation Elevator/1 -> Sum4/1, Mux/1
  Sum4/1 -> anti windup/1
  anti windup/1 -> Sum9/1
  phi controller integrator/1 -> Sum/2
  Sum/1 -> Saturation Aileron/1, Sum6/1
  Demux4/3 -> Mux/3  "throttle"
  attitude demands/1 -> Demux4/1  "theta_d phi_d tau_d"
  Mux/1 -> demands/1  "eta_d xi_d tau_d"
  Demux4/1 -> Sum3/1  "theta_d"
  Attitude PI Controller - Bank Angle to Aileron/1 -> Sum/1
  Demux2/2 -> Terminator2/1  "earthspeed"
  Demux2/3 -> Terminator1/1  "measured acceleration"
  Sensors/1 -> Demux2/1
  Demux2/5 -> Terminator4/1  "t qbar P"
  Demux2/1 -> Terminator/1  "position"
  Demux2/6 -> Demux1/1  "attitude"
  Demux1/1 -> Sum1/2  "phi"
  Demux1/2 -> Sum3/2  "theta"
  Demux1/3 -> Terminator5/1  "psi"
  Demux2/4 -> Terminator6/1  "rates"
  Saturation Aileron/1 -> Mux/2, Sum6/2
  Gain1/1 -> Sum5/1
  Sum5/1 -> phi controller integrator/1
  Sum6/1 -> Sum5/2

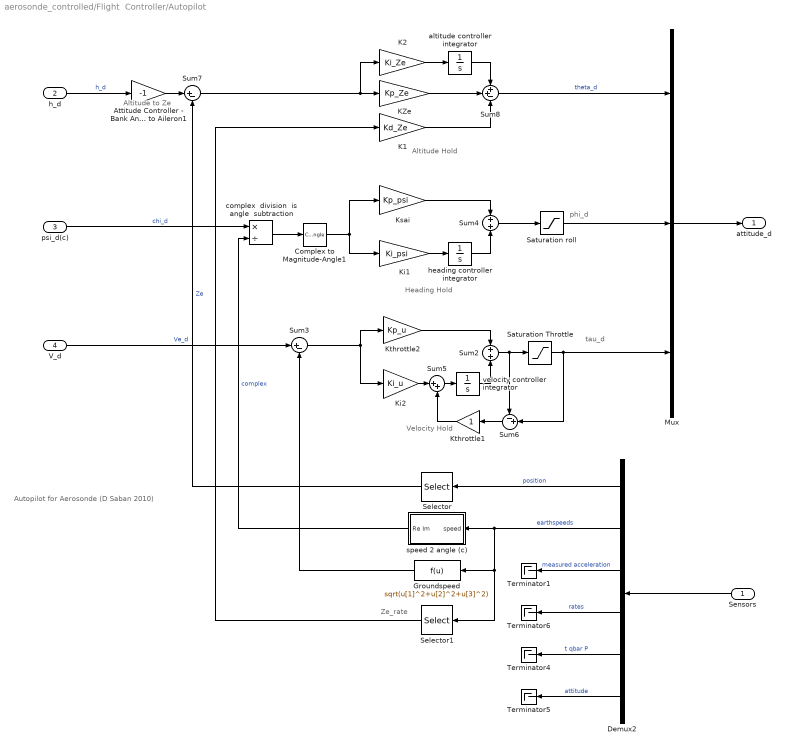
== system aerosonde_controlled/Flight  Controller/Autopilot ==
  note: Heading Hold
  note: Altitude to Ze
  note: Velocity Hold
  note: Altitude Hold
  note: phi_d
  note: tau_d
  note: Ze_rate
  note: Autopilot
      | for Aerosonde
      | (D Saban 2010)
  Sensors : Inport
  h_d : Inport  Port=2
  psi_d(c) : Inport  Port=3
  V_d : Inport  Port=4
  Attitude Controller - Bank Angle to Aileron1 : Gain  Gain=-1
  Complex to Magnitude-Angle1 : ComplexToMagnitudeAngle  Output=Angle
  Demux2 : Demux  Outputs=[3 3 3 3 3 3]
  Groundspeed : Fcn  Expr=sqrt(u[1]^2+u[2]^2+u[3]^2)
  K1 : Gain  Gain=Kd_Ze
  K2 : Gain  Gain=Ki_Ze
  KZe : Gain  Gain=Kp_Ze
  Ki1 : Gain  Gain=Ki_psi
  Ki2 : Gain  Gain=Ki_u
  Ksai : Gain  Gain=Kp_psi
  Kthrottle1 : Gain
  Kthrottle2 : Gain  Gain=Kp_u
  Mux : Mux  Inputs=3
  Saturation Throttle : Saturate  UpperLimit=1  LowerLimit=0  ZeroCross=off
  Saturation roll : Saturate  UpperLimit=1.1  LowerLimit=-1.1  ZeroCross=off
  Selector : Selector  InputPortWidth=3  IndexOptions=Index vector (dialog)  Indices=3  OutputSizes=1
  Selector1 : Selector  InputPortWidth=3  IndexOptions=Index vector (dialog)  Indices=3  OutputSizes=1
  Sum2 : Sum
  Sum3 : Sum  Inputs=|+-
  Sum4 : Sum
  Sum5 : Sum  Inputs=|++
  Sum6 : Sum  Inputs=-+|
  Sum7 : Sum  Inputs=|+-
  Sum8 : Sum  Inputs=++-
  Terminator{1,4..6} (4 alike) : Terminator
  altitude controller integrator : Integrator  InitialCondition=theta_trim  LimitOutput=on  UpperSaturationLimit=.3  LowerSaturationLimit=-.3
  complex  division  is angle  subtraction : Product  Inputs=*/
  heading controller integrator : Integrator  InitialCondition=chi_trim  LimitOutput=on  UpperSaturationLimit=1.2  LowerSaturationLimit=-1.2
  speed 2 angle (c) : Subsystem
  velocity controller integrator : Integrator  InitialCondition=tau_trim
  attitude_d : Outport
  wires:
  Ksai/1 -> Sum4/1
  Sum7/1 -> KZe/1, K2/1
  KZe/1 -> Sum8/2
  K2/1 -> altitude controller integrator/1
  altitude controller integrator/1 -> Sum8/1
  K1/1 -> Sum8/3
  Attitude Controller - Bank Angle to Aileron1/1 -> Sum7/1
  Kthrottle2/1 -> Sum2/1
  Sum2/1 -> Saturation Throttle/1, Sum6/1
  Sum3/1 -> Kthrottle2/1, Ki2/1
  Saturation Throttle/1 -> Sum6/2, Mux/3
  Ki2/1 -> Sum5/1
  Sum5/1 -> velocity controller integrator/1
  velocity controller integrator/1 -> Sum2/2
  Sum6/1 -> Kthrottle1/1
  Kthrottle1/1 -> Sum5/2
  Ki1/1 -> heading controller integrator/1
  h_d/1 -> Attitude Controller - Bank Angle to Aileron1/1  "h_d"
  V_d/1 -> Sum3/1  "Ve_d"
  Sum8/1 -> Mux/1  "theta_d"
  Sum4/1 -> Saturation roll/1
  Demux2/2 -> Groundspeed/1, Selector1/1, speed 2 angle (c)/1(speed)  "earthspeeds"
  Demux2/3 -> Terminator1/1  "measured acceleration"
  Sensors/1 -> Demux2/1
  Demux2/5 -> Terminator4/1  "t qbar P"
  Demux2/1 -> Selector/1  "position"
  Demux2/4 -> Terminator6/1  "rates"
  Demux2/6 -> Terminator5/1  "attitude"
  Selector/1 -> Sum7/2  "Ze"
  Groundspeed/1 -> Sum3/2
  heading controller integrator/1 -> Sum4/2
  Selector1/1 -> K1/1
  Mux/1 -> attitude_d/1
  psi_d(c)/1 -> complex  division  is angle  subtraction/1  "chi_d"
  Saturation roll/1 -> Mux/2
  speed 2 angle (c)/1(Re Im) -> complex  division  is angle  subtraction/2  "complex"
  complex  division  is angle  subtraction/1 -> Complex to Magnitude-Angle1/1
  Complex to Magnitude-Angle1/1 -> Ksai/1, Ki1/1

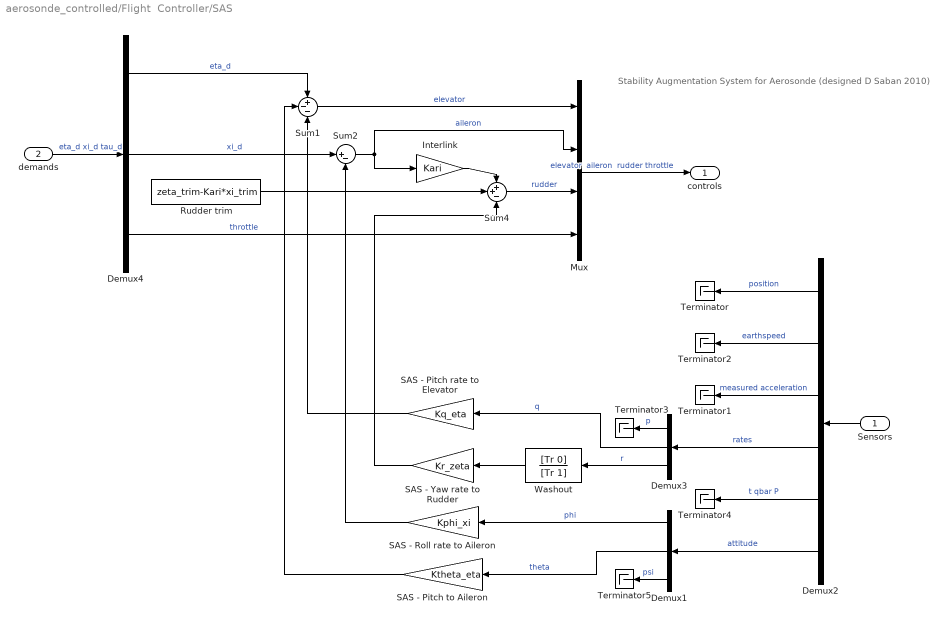
== system aerosonde_controlled/Flight  Controller/SAS ==
  note: Stability Augmentation System
      | for Aerosonde
      | (designed D Saban 2010)
  Sensors : Inport
  demands : Inport  Port=2
  Demux1 : Demux  Outputs=3
  Demux2 : Demux  Outputs=[3 3 3 3 3 3]
  Demux3 : Demux  Outputs=3
  Demux4 : Demux  Outputs=3
  Interlink : Gain  Gain=Kari
  Mux : Mux
  Rudder trim : Constant  Value=zeta_trim-Kari*xi_trim
  SAS - Pitch rate to Elevator : Gain  Gain=Kq_eta
  SAS - Pitch to Aileron : Gain  Gain=Ktheta_eta
  SAS - Roll rate to Aileron : Gain  Gain=Kphi_xi
  SAS - Yaw rate to Rudder : Gain  Gain=Kr_zeta
  Sum1 : Sum  Inputs=+--
  Sum2 : Sum  Inputs=|+-
  Sum4 : Sum  Inputs=++-
  Terminator{,1..5} (6 alike) : Terminator
  Washout : TransferFcn  Numerator=[Tr 0]  Denominator=[Tr 1]
  controls : Outport
  wires:
  Washout/1 -> SAS - Yaw rate to Rudder/1
  Demux3/3 -> Washout/1  "r"
  Demux2/2 -> Terminator2/1  "earthspeed"
  Demux2/3 -> Terminator1/1  "measured acceleration"
  Sensors/1 -> Demux2/1
  Demux2/4 -> Demux3/1  "rates"
  Demux2/5 -> Terminator4/1  "t qbar P"
  Demux3/2 -> SAS - Pitch rate to Elevator/1  "q"
  Demux2/1 -> Terminator/1  "position"
  Demux2/6 -> Demux1/1  "attitude"
  Demux3/1 -> Terminator3/1  "p"
  Demux4/3 -> Mux/4  "throttle"
  Sum4/1 -> Mux/3  "rudder"
  Sum1/1 -> Mux/1  "elevator"
  Demux4/1 -> Sum1/1  "eta_d"
  Demux4/2 -> Sum2/1  "xi_d"
  Sum2/1 -> Interlink/1, Mux/2  "aileron"
  Rudder trim/1 -> Sum4/2
  Interlink/1 -> Sum4/1
  Demux1/1 -> SAS - Roll rate to Aileron/1  "phi"
  Demux1/2 -> SAS - Pitch to Aileron/1  "theta"
  SAS - Pitch to Aileron/1 -> Sum1/2
  Demux1/3 -> Terminator5/1  "psi"
  SAS - Yaw rate to Rudder/1 -> Sum4/3
  SAS - Roll rate to Aileron/1 -> Sum2/2
  SAS - Pitch rate to Elevator/1 -> Sum1/3
  Mux/1 -> controls/1  "elevator  aileron  rudder throttle"
  demands/1 -> Demux4/1  "eta_d xi_d tau_d"
